simulink model "Hysteresis_Experiment_SimScape"  (R2018b)
settings: Solver=VariableStepAuto  StartTime=0.0  StopTime=10  RelTol=1e-3
libraries: fl_lib x4, nesl_utility x4, Non_ideal_memristor_resistances_lib x1, simulink x1
settings Model: Creator=dsentc  LastModifiedBy=poker
settings DebuggingCC: LibraryContextMissingDiagnostic=none
settings SFSimCC: SimUseLocalCustomCode=off
settings RTWCC: RTWUseLocalCustomCode=off

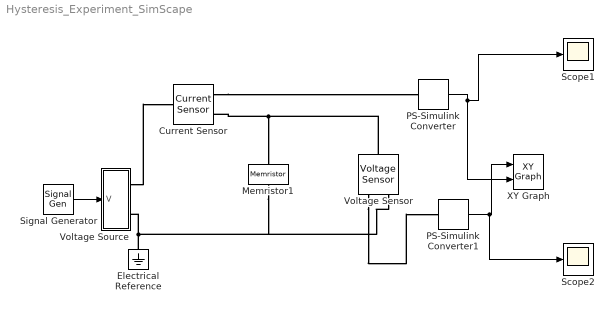
== system Hysteresis_Experiment_SimScape ==
  Current Sensor : fl_lib/Electrical/Electrical Sensors/Current Sensor
  Electrical Reference : fl_lib/Electrical/Electrical Elements/Electrical Reference
  Memristor1 : Non_ideal_memristor_resistances_lib/Memristor  Ra=1341 Ohm  Rb=111355 Ohm  Q0=1e-2 C  x0=0.1  pwindow=2  i_specify=off  i_priority=None  i=0 A  i_nominal_specify=off  i_nominal_unit=A  i_nominal_value=1  v_specify=off  v_priority=None  v=0 V  v_nominal_specify=off  v_nominal_unit=V  v_nominal_value=1
  PS-Simulink Converter : nesl_utility/PS-Simulink Converter  PhysicalDomain=network_engine_domain  SubClassName=ps_output  LeftPortType=input  RightPortType=output  PseudoPeriodic=off  Frequencies=[]  Unit=1  AffineConversion=off
  PS-Simulink Converter1 : nesl_utility/PS-Simulink Converter  PhysicalDomain=network_engine_domain  SubClassName=ps_output  LeftPortType=input  RightPortType=output  PseudoPeriodic=off  Frequencies=[]  Unit=1  AffineConversion=off
  Scope1 : Scope
  Scope2 : Scope
  Signal Generator : SignalGenerator  Amplitude=5  Frequency=.1592
  Voltage Source : Subsystem
  Voltage Sensor : fl_lib/Electrical/Electrical Sensors/Voltage Sensor
  XY Graph : simulink/Sinks/XY Graph  xmin=-5  xmax=5  ymin=-1  ymax=1  st=-1
  wires:
  Signal Generator/1 -> Voltage Source/1(V)
  PS-Simulink Converter1/1 -> Scope2/1, XY Graph/1
  PS-Simulink Converter/1 -> Scope1/1, XY Graph/2
  connections:
  Electrical Reference/LConn1 -- Memristor1/LConn1 -- Voltage Sensor/RConn2 -- Voltage Source/RConn2
  Voltage Source/RConn1 -- Current Sensor/LConn1
  Voltage Sensor/LConn1 -- Memristor1/RConn1 -- Current Sensor/RConn2
  Current Sensor/RConn1 -- PS-Simulink Converter/LConn1
  Voltage Sensor/RConn1 -- PS-Simulink Converter1/LConn1

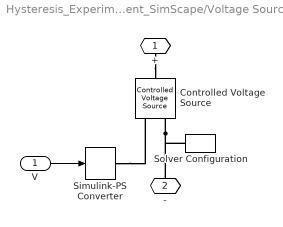
== system Hysteresis_Experiment_SimScape/Voltage Source ==
  V : Inport
  Controlled Voltage Source : fl_lib/Electrical/Electrical Sources/Controlled Voltage Source
  Simulink-PS Converter : nesl_utility/Simulink-PS Converter  PhysicalDomain=network_engine_domain  SubClassName=ps_input  LeftPortType=input  RightPortType=output  PseudoPeriodic=off  Frequencies=[]  NoiseDistribution=none  NoiseParameters=[]  Unit=1  AffineConversion=off  FilteringAndDerivatives=zero  SimscapeFilterOrder=1  InputFilterTimeConstant=.001  UdotUserProvided=0
  Solver Configuration : nesl_utility/Solver Configuration  PhysicalDomain=network_engine_domain  SubClassName=solver  LeftPortType=input  RightPortType=generic  Tones=[]  Harmonics=[]  SimulateNoise=off  Profile=off  UseLocalSampling=off  EnableSwitchedLinearOptims=on  FrequencyDomain=off  UseCCode=off  RelTol=0.001  AbsTol=1e-06  MinStep=1e-09  ToWorkspace=off  RevertToSquareIcSolve=off  NumHomotopyIterations=100  PhasorMode=off  PhasorModeNumHarmonics=1  DoDC=off  ResidualTolerance=1e-9  UseLocalSolver=off  LocalSolverChoice=NE_BACKWARD_EULER_ADVANCER  LocalSolverSampleTime=.001  DoFixedCost=off  MaxNonlinIter=3  MaxModeIter=2  LinearAlgebra=Full  EquationFormulation=NE_TIME_EF  DelaysMemoryBudget=1024  AutomaticFiltering=on  FilteringTimeConstant=0.00001  PartitionStorageMethod=AS_NEEDED  PartitionMemoryBudget=1024
  + : PMIOPort  Side=Right
  - : PMIOPort  Port=2  Side=Right
  wires:
  V/1 -> Simulink-PS Converter/1
  connections:
  Simulink-PS Converter/RConn1 -- Controlled Voltage Source/RConn1
  Controlled Voltage Source/RConn2 -- -/RConn1 -- Solver Configuration/RConn1
  +/RConn1 -- Controlled Voltage Source/LConn1
